simulink model "early_exit"  (R2018a)
settings: Solver=VariableStepAuto  StartTime=0.0  StopTime=10.0  RelTol=1e-3
settings Model: Creator=BEAR  LastModifiedBy=BEAR

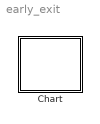
== system early_exit ==
  Chart : Stateflow chart  TreatAsAtomicUnit=on

== stateflow chart early_exit/Chart ==
  state A
    state A1
    state A2
    (default) -> A1
    A1 -> A2 : {e}
  state B
  (default) -> A
  A -> B : e
  events: e local FUNCTION_CALL_EVENT
